simulink model "Triggered1_2018a"  (R2018a)
settings: Solver=VariableStepAuto  StartTime=0.0  StopTime=5  RelTol=1e-3
settings Model: Creator=BEAR  LastModifiedBy=bzhan

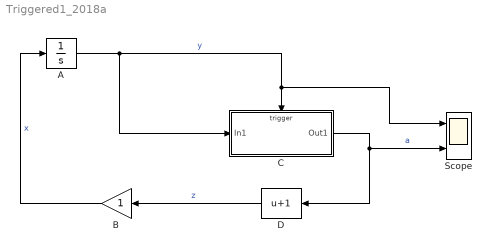
== system Triggered1_2018a ==
  A : Integrator  InitialCondition=-1
  B : Gain  SampleTime=1
  C : Subsystem  TreatAsAtomicUnit=on
  D : Bias  Bias=1
  Scope : Scope  NumInputPorts=2
  wires:
  C/1(Out1) -> Scope/2, D/1  "a"
  A/1 -> Scope/1, C/Trigger, C/1(In1)  "y"
  D/1 -> B/1  "z"
  B/1 -> A/1  "x"

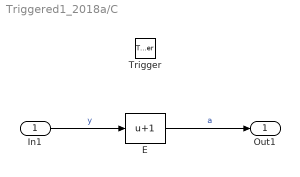
== system Triggered1_2018a/C ==
  In1 : Inport
  Trigger : TriggerPort  VariantControl=Variant
  E : Bias  Bias=1
  Out1 : Outport  VectorParamsAs1DForOutWhenUnconnected=off
  wires:
  E/1 -> Out1/1  "a"
  In1/1 -> E/1  "y"
